simulink model "b_r309c_med"  (Simulink 6.2)
settings: Solver=ode45  StartTime=0.0  StopTime=1030.0  RelTol=1e-3
undefined symbols (not defined in the file): ant_bits, BEE2_usr, blockCountBits, blockRowBits, cmult_4bit_em
libraries: xbsIndex_r3 x2808, xps_library x97, casper_library x84
(part 7 of 20)

== system b_r309c_med/fmt_for_dram0/mk_4x32bit ==
  din : Inport  Port=1  LatchInput=off
  Concat3 : xbsIndex_r3/Concat  num_inputs=4  explicit_period=off  period=1  dbl_ovrd=off
  Convert{1..4} (4 alike) : xbsIndex_r3/Convert  arith_type="Signed  (2's comp)"  n_bits=32  bin_pt=0  quantization=Truncate  overflow=Wrap  latency=0  explicit_period=off  period=1  dbl_ovrd=off  show_param=off  inserted_by_tool=off  pipeline=off
      settings: xl_area=[0, 0, 0, 0, 0, 0, 0]
  Gateway Out{1..4,13..16} (8 alike) : xbsIndex_r3/Gateway Out  output_type=Double  nbits=8  bin_pt=6  arith_type=Boolean  quantization=Truncate  overflow=Wrap  hdl_port=off  timing_constraint=None  locs_specified=off  LOCs={}  needs_fixed_name=off  show_param=off
      settings: xl_area=[0, 0, 0, 0, 0, 0, 0]
  Reinterpret{,2,4,6} (4 alike) : xbsIndex_r3/Reinterpret  force_arith_type=on  arith_type=Unsigned  force_bin_pt=on  bin_pt=0  force_valid=on
  Reinterpret{1,3,5,7} (4 alike) : xbsIndex_r3/Reinterpret  force_arith_type=on  arith_type="Signed  (2's comp)"  force_bin_pt=on  bin_pt=0  force_valid=on
  Scope2 : Scope  NumInputPorts=8
      settings: YMin=0~0~0~0~0~0~0~0  YMax=20~20~20~20~20~20~20~20  SaveName=ScopeData3
  Slice10 : xbsIndex_r3/Slice  mode=Lower Bit Location + Width  nbits=(2*x_n_bits+1+x_int_bits)  bit1=0  base1=MSB of Input  bit0=2*(2*x_n_bits+1+x_int_bits)  base0=LSB of Input  boolean_output=off  explicit_period=off  period=1  dbl_ovrd=off
  Slice11 : xbsIndex_r3/Slice  mode=Lower Bit Location + Width  nbits=(2*x_n_bits+1+x_int_bits)  bit1=0  base1=MSB of Input  bit0=0  base0=LSB of Input  boolean_output=off  explicit_period=off  period=1  dbl_ovrd=off
  Slice12 : xbsIndex_r3/Slice  mode=Lower Bit Location + Width  nbits=(2*x_n_bits+1+x_int_bits)  bit1=0  base1=MSB of Input  bit0=(2*x_n_bits+1+x_int_bits)  base0=LSB of Input  boolean_output=off  explicit_period=off  period=1  dbl_ovrd=off
  Slice7 : xbsIndex_r3/Slice  mode=Lower Bit Location + Width  nbits=(2*x_n_bits+1+x_int_bits)  bit1=0  base1=MSB of Input  bit0=3*(2*x_n_bits+1+x_int_bits)  base0=LSB of Input  boolean_output=off  explicit_period=off  period=1  dbl_ovrd=off
  dout : Outport
  wires:
  Concat3/1 -> dout/1
  din/1 -> Slice12/1, Slice11/1, Slice10/1, Slice7/1
  Reinterpret6/1 -> Concat3/4
  Reinterpret4/1 -> Concat3/3
  Reinterpret2/1 -> Concat3/2
  Convert4/1 -> Reinterpret6/1, Gateway Out1/1
  Reinterpret7/1 -> Convert4/1, Gateway Out4/1
  Slice11/1 -> Reinterpret7/1
  Convert3/1 -> Reinterpret4/1, Gateway Out3/1
  Reinterpret5/1 -> Convert3/1, Gateway Out2/1
  Slice12/1 -> Reinterpret5/1
  Convert2/1 -> Reinterpret2/1, Gateway Out13/1
  Reinterpret3/1 -> Convert2/1, Gateway Out16/1
  Slice10/1 -> Reinterpret3/1
  Reinterpret/1 -> Concat3/1
  Convert1/1 -> Reinterpret/1, Gateway Out15/1
  Reinterpret1/1 -> Convert1/1, Gateway Out14/1
  Slice7/1 -> Reinterpret1/1
  Gateway Out14/1 -> Scope2/1
  Gateway Out15/1 -> Scope2/2
  Gateway Out16/1 -> Scope2/3
  Gateway Out13/1 -> Scope2/4
  Gateway Out2/1 -> Scope2/5
  Gateway Out3/1 -> Scope2/6
  Gateway Out4/1 -> Scope2/7
  Gateway Out1/1 -> Scope2/8

== system b_r309c_med/loopback0/fwft_fifo ==
  din : Inport  Port=1  LatchInput=off
  we : Inport  Port=2  LatchInput=off
  ack : Inport  Port=3  LatchInput=off
  Convert : xbsIndex_r3/Convert  Orientation=left  arith_type=Boolean  n_bits=1  bin_pt=0  quantization=Truncate  overflow=Wrap  latency=0  explicit_period=off  period=1  dbl_ovrd=off  show_param=off  inserted_by_tool=off  pipeline=off
      settings: xl_area=[0, 0, 0, 0, 0, 0, 0]
  FIFO : xbsIndex_r3/FIFO  depth=256  percent_nbits=1  store_only_valid=on  init_zero=on  explicit_period=off  period=1  rst=off  en=off  use_almost_empty=off  almost_empty_offset=6  use_almost_full=off  almost_full_offset=6  dbl_ovrd=off  show_param=off  mem_type=Block RAM  gen_core=off
      settings: xl_area=[0, 0, 0, 0, 0, 0, 0]
  Inverter1 : xbsIndex_r3/Inverter  latency=0  explicit_period=off  period=1  en=off  dbl_ovrd=off  show_param=off
      settings: xl_area=[0, 0, 0, 0, 0, 0, 0]
  Logical1 : xbsIndex_r3/Logical  logical_function=OR  inputs=2  precision=Full  arith_type=Unsigned  n_bits=8  bin_pt=2  align_bp=on  latency=0  explicit_period=off  period=1  en=off  dbl_ovrd=off  show_param=off
      settings: xl_area=[0, 0, 0, 0, 0, 0, 0]
  Register2 : xbsIndex_r3/Register  init=0  reg_only_valid=off  explicit_period=on  period=1  rst=off  en=on  out_en=off  dbl_ovrd=off  show_param=off
      settings: xl_area=[0, 0, 0, 0, 0, 0, 0]
  dout : Outport
  valid : Outport  Port=2
  wires:
  din/1 -> FIFO/1
  we/1 -> FIFO/2
  FIFO/1 -> dout/1
  FIFO/2 -> Register2/1
  Logical1/1 -> FIFO/3, Register2/2
  ack/1 -> Logical1/1
  Register2/1 -> Convert/1, Inverter1/1
  Convert/1 -> Logical1/2
  Inverter1/1 -> valid/1

== system b_r309c_med/loopback0/rollback_fifo ==
  din : Inport  Port=1  LatchInput=off
  we : Inport  Orientation=left  Port=2  LatchInput=off
  commit : Inport  Port=3  LatchInput=off
  discard : Inport  Port=4  LatchInput=off
  re : Inport  Port=5  LatchInput=off
  Constant5 : xbsIndex_r3/Constant  const=0  equ=P=C  arith_type=Boolean  n_bits=1  bin_pt=0  opselect=C  inp2=PCIN>>17  opr=+  inp1=P  carry=CIN  iostate=0  explicit_period=on  period=1  dbl_ovrd=off
  Delay1 : xbsIndex_r3/Delay  latency=1  reg_retiming=off  explicit_period=off  period=1  en=off  accept_only_valid=off  init_zero=on  dbl_ovrd=off  show_param=off
      settings: xl_area=[0, 0, 0, 0, 0, 0, 0]
  Dual Port RAM : xbsIndex_r3/Dual Port RAM  depth=2^depth_bits  initVector=0  write_mode_A=Read Before Write  write_mode_B=Read Before Write  latency=1  mem_collision=off  init_zero=on  explicit_period=off  period=1  dbl_ovrd=off  rst_a=off  init_a=0  rst_b=off  init_b=0  show_param=off  distributed_mem=off  use_rpm=off  gen_core=off
      settings: xl_area=[0, 0, 0, 0, 0, 0, 0]
  Inverter1 : xbsIndex_r3/Inverter  latency=0  explicit_period=off  period=1  en=off  dbl_ovrd=off  show_param=off
      settings: xl_area=[0, 0, 0, 0, 0, 0, 0]
  Inverter2 : xbsIndex_r3/Inverter  Orientation=up  latency=0  explicit_period=off  period=1  en=off  dbl_ovrd=off  show_param=off
      settings: xl_area=[0, 0, 0, 0, 0, 0, 0]
  Logical1 : xbsIndex_r3/Logical  logical_function=AND  inputs=2  precision=Full  arith_type=Unsigned  n_bits=8  bin_pt=2  align_bp=on  latency=0  explicit_period=off  period=1  en=off  dbl_ovrd=off  show_param=off
      settings: xl_area=[0, 0, 0, 0, 0, 0, 0]
  Logical3 : xbsIndex_r3/Logical  Orientation=left  logical_function=AND  inputs=2  precision=Full  arith_type=Unsigned  n_bits=8  bin_pt=2  align_bp=on  latency=0  explicit_period=off  period=1  en=off  dbl_ovrd=off  show_param=off
      settings: xl_area=[0, 0, 0, 0, 0, 0, 0]
  Logical4 : xbsIndex_r3/Logical  logical_function=AND  inputs=2  precision=Full  arith_type=Unsigned  n_bits=8  bin_pt=2  align_bp=on  latency=0  explicit_period=off  period=1  en=off  dbl_ovrd=off  show_param=off
      settings: xl_area=[0, 0, 0, 0, 0, 0, 0]
  Logical5 : xbsIndex_r3/Logical  logical_function=XOR  inputs=2  precision=Full  arith_type=Unsigned  n_bits=8  bin_pt=2  align_bp=on  latency=0  explicit_period=off  period=1  en=off  dbl_ovrd=off  show_param=off
      settings: xl_area=[0, 0, 0, 0, 0, 0, 0]
  Logical6 : xbsIndex_r3/Logical  logical_function=AND  inputs=2  precision=Full  arith_type=Unsigned  n_bits=8  bin_pt=2  align_bp=on  latency=0  explicit_period=off  period=1  en=off  dbl_ovrd=off  show_param=off
      settings: xl_area=[0, 0, 0, 0, 0, 0, 0]
  Relational1 : xbsIndex_r3/Relational  mode=a=b  latency=0  explicit_period=on  period=1  en=off  dbl_ovrd=off  show_param=off
      settings: xl_area=[0, 0, 0, 0, 0, 0, 0]
  Relational2 : xbsIndex_r3/Relational  mode=a=b  latency=0  explicit_period=on  period=1  en=off  dbl_ovrd=off  show_param=off
      settings: xl_area=[0, 0, 0, 0, 0, 0, 0]
  Slice : xbsIndex_r3/Slice  mode=Two Bit Locations  nbits=1  bit1=-1  base1=MSB of Input  bit0=0  base0=LSB of Input  boolean_output=off  explicit_period=off  period=1  dbl_ovrd=off
  Slice1 : xbsIndex_r3/Slice  mode=Upper Bit Location + Width  nbits=1  bit1=0  base1=MSB of Input  bit0=0  base0=LSB of Input  boolean_output=on  explicit_period=off  period=1  dbl_ovrd=off
  Slice2 : xbsIndex_r3/Slice  mode=Two Bit Locations  nbits=1  bit1=-1  base1=MSB of Input  bit0=0  base0=LSB of Input  boolean_output=off  explicit_period=off  period=1  dbl_ovrd=off
  Slice3 : xbsIndex_r3/Slice  mode=Upper Bit Location + Width  nbits=1  bit1=0  base1=MSB of Input  bit0=0  base0=LSB of Input  boolean_output=on  explicit_period=off  period=1  dbl_ovrd=off
  rd_cnt : xbsIndex_r3/Counter  cnt_type=Free Running  n_bits=depth_bits + 1  bin_pt=0  arith_type=Unsigned  start_count=0  cnt_to=Inf  cnt_by_val=1  operation=Up  explicit_period=on  period=1  load_pin=off  rst=off  en=on  dbl_ovrd=off  show_param=off  use_rpm=on  gen_core=off
      settings: xl_area=[0, 0, 0, 0, 0, 0, 0]
  set_cnt : Subsystem
  dout : Outport
  valid : Outport  Port=2
  wr_ack : Outport  Orientation=left  Port=3
  full : Outport  Port=4
  empty : Outport  Port=5
  wires:
  Relational2/1 -> Logical1/1
  Logical6/1 -> Inverter2/1, full/1
  Logical5/1 -> Logical6/1
  Relational1/1 -> Logical6/2
  Slice1/1 -> Logical5/2
  Slice3/1 -> Logical5/1
  Slice2/1 -> Relational1/1, Dual Port RAM/1
  din/1 -> Dual Port RAM/2, Dual Port RAM/5
  Slice/1 -> Relational1/2, Dual Port RAM/4
  set_cnt/2(cnt) -> Slice2/1, Slice3/1
  set_cnt/1(set_cnt) -> Relational2/1
  rd_cnt/1 -> Relational2/2, Slice1/1, Slice/1
  commit/1 -> set_cnt/1(set)
  Inverter2/1 -> Logical1/2, Logical3/1
  we/1 -> Logical3/2
  Logical3/1 -> wr_ack/1, Dual Port RAM/3, set_cnt/3(en)
  discard/1 -> set_cnt/2(undo)
  Constant5/1 -> Dual Port RAM/6
  Dual Port RAM/2 -> dout/1
  Logical1/1 -> Inverter1/1, empty/1
  Inverter1/1 -> Logical4/2
  re/1 -> Logical4/1
  Logical4/1 -> rd_cnt/1, Delay1/1
  Delay1/1 -> valid/1

== system b_r309c_med/mux_pkts0/state_mach ==
  note: state
  note: output
  gbe_valid : Inport  Port=1  LatchInput=off
  pkt_rdy : Inport  Port=2  LatchInput=off
  eof : Inport  Port=3  LatchInput=off
  Constant4 : xbsIndex_r3/Constant  const=1  equ=P=C  arith_type=Boolean  n_bits=1  bin_pt=0  opselect=C  inp2=PCIN>>17  opr=+  inp1=P  carry=CIN  iostate=0  explicit_period=on  period=1  dbl_ovrd=off
  Convert : xbsIndex_r3/Convert  arith_type=Boolean  n_bits=8  bin_pt=6  quantization=Truncate  overflow=Wrap  latency=0  explicit_period=off  period=1  dbl_ovrd=off  show_param=off  inserted_by_tool=off  pipeline=off
      settings: xl_area=[0, 0, 0, 0, 0, 0, 0]
  Inverter : xbsIndex_r3/Inverter  latency=0  explicit_period=off  period=1  en=off  dbl_ovrd=off  show_param=off
      settings: xl_area=[0, 0, 0, 0, 0, 0, 0]
  Inverter1 : xbsIndex_r3/Inverter  Orientation=left  latency=0  explicit_period=off  period=1  en=off  dbl_ovrd=off  show_param=off
      settings: xl_area=[0, 0, 0, 0, 0, 0, 0]
  Inverter2 : xbsIndex_r3/Inverter  latency=0  explicit_period=off  period=1  en=off  dbl_ovrd=off  show_param=off
      settings: xl_area=[0, 0, 0, 0, 0, 0, 0]
  Logical1 : xbsIndex_r3/Logical  logical_function=AND  inputs=2  precision=Full  arith_type=Unsigned  n_bits=8  bin_pt=2  align_bp=on  latency=0  explicit_period=off  period=1  en=off  dbl_ovrd=off  show_param=off
      settings: xl_area=[0, 0, 0, 0, 0, 0, 0]
  Logical2 : xbsIndex_r3/Logical  logical_function=OR  inputs=2  precision=Full  arith_type=Unsigned  n_bits=8  bin_pt=2  align_bp=on  latency=0  explicit_period=off  period=1  en=off  dbl_ovrd=off  show_param=off
      settings: xl_area=[0, 0, 0, 0, 0, 0, 0]
  Logical3 : xbsIndex_r3/Logical  logical_function=AND  inputs=2  precision=Full  arith_type=Unsigned  n_bits=8  bin_pt=2  align_bp=on  latency=0  explicit_period=off  period=1  en=off  dbl_ovrd=off  show_param=off
      settings: xl_area=[0, 0, 0, 0, 0, 0, 0]
  Logical4 : xbsIndex_r3/Logical  logical_function=AND  inputs=2  precision=Full  arith_type=Unsigned  n_bits=8  bin_pt=2  align_bp=on  latency=0  explicit_period=off  period=1  en=off  dbl_ovrd=off  show_param=off
      settings: xl_area=[0, 0, 0, 0, 0, 0, 0]
  Register1 : xbsIndex_r3/Register  init=0  reg_only_valid=off  explicit_period=on  period=1  rst=on  en=on  out_en=off  dbl_ovrd=off  show_param=off
      settings: xl_area=[0, 0, 0, 0, 0, 0, 0]
  Register2 : xbsIndex_r3/Register  init=0  reg_only_valid=off  explicit_period=on  period=1  rst=off  en=on  out_en=off  dbl_ovrd=off  show_param=off
      settings: xl_area=[0, 0, 0, 0, 0, 0, 0]
  gbe_ack : Outport
  loop_ack : Outport  Port=2
  state : Outport  Port=3
  wires:
  Register1/1 -> Convert/1
  Constant4/1 -> Register1/1
  Logical2/1 -> Logical3/2, Register1/3
  Logical3/1 -> Register2/2
  Inverter2/1 -> Register2/1
  gbe_valid/1 -> Logical2/1
  Register2/1 -> Inverter/1, Logical4/2
  Inverter1/1 -> Logical3/1
  eof/1 -> Register1/2
  Inverter/1 -> Logical1/2
  Logical1/1 -> loop_ack/1
  Logical4/1 -> gbe_ack/1
  pkt_rdy/1 -> Logical2/2, Inverter2/1
  Convert/1 -> state/1, Logical1/1, Logical4/1, Inverter1/1

== system b_r309c_med/out_mon0/stopwatch ==
  stop : Inport  Port=1  LatchInput=off
  start : Inport  Port=2  LatchInput=off
  reset : Inport  Port=3  LatchInput=off
  count : Inport  Port=4  LatchInput=off
  Constant1 : xbsIndex_r3/Constant  const=1  equ=P=C  arith_type=Boolean  n_bits=1  bin_pt=0  opselect=C  inp2=PCIN>>17  opr=+  inp1=P  carry=CIN  iostate=0  explicit_period=on  period=1  dbl_ovrd=off
  Constant8 : xbsIndex_r3/Constant  const=1  equ=P=C  arith_type=Boolean  n_bits=1  bin_pt=0  opselect=C  inp2=PCIN>>17  opr=+  inp1=P  carry=CIN  iostate=0  explicit_period=on  period=1  dbl_ovrd=off
  Counter1 : xbsIndex_r3/Counter  cnt_type=Free Running  n_bits=32  bin_pt=0  arith_type=Unsigned  start_count=0  cnt_to=Inf  cnt_by_val=1  operation=Up  explicit_period=off  period=1  load_pin=off  rst=on  en=on  dbl_ovrd=off  show_param=off  use_rpm=on  gen_core=off
      settings: xl_area=[0, 0, 0, 0, 0, 0, 0]
  Logical : xbsIndex_r3/Logical  logical_function=AND  inputs=3  precision=Full  arith_type=Unsigned  n_bits=8  bin_pt=2  align_bp=on  latency=0  explicit_period=off  period=1  en=off  dbl_ovrd=off  show_param=off
      settings: xl_area=[0, 0, 0, 0, 0, 0, 0]
  Register1 : xbsIndex_r3/Register  init=0  reg_only_valid=off  explicit_period=off  period=1  rst=on  en=on  out_en=off  dbl_ovrd=off  show_param=off
      settings: xl_area=[0, 0, 0, 0, 0, 0, 0]
  Register3 : xbsIndex_r3/Register  init=0  reg_only_valid=off  explicit_period=off  period=1  rst=on  en=on  out_en=off  dbl_ovrd=off  show_param=off
      settings: xl_area=[0, 0, 0, 0, 0, 0, 0]
  count_out : Outport
  wires:
  Constant8/1 -> Register3/1
  Counter1/1 -> count_out/1
  Constant1/1 -> Register1/1
  start/1 -> Register1/3
  reset/1 -> Counter1/1, Register1/2, Register3/3
  Logical/1 -> Counter1/2
  Register3/1 -> Logical/1
  Register1/1 -> Logical/2
  stop/1 -> Register3/2
  count/1 -> Logical/3

== system b_r309c_med/out_mon0/x_eng_cntr ==
  note: n_ants*(n_ants+1)/2 * n_chans/n_xeng-1
  acc_in : Inport  Port=1  LatchInput=off
  valid_in : Inport  Port=2  LatchInput=off
  sync_in : Inport  Port=3  LatchInput=off
  Constant9 : xbsIndex_r3/Constant  Orientation=left  const=n_ants*(n_ants+1)/2 * n_chans/n_xeng-1  equ=P=C  arith_type=Unsigned  n_bits=32  bin_pt=0  opselect=C  inp2=PCIN>>17  opr=+  inp1=P  carry=CIN  iostate=0  explicit_period=on  period=1  dbl_ovrd=off
  Logical6 : xbsIndex_r3/Logical  logical_function=OR  inputs=2  precision=Full  arith_type=Unsigned  n_bits=8  bin_pt=2  align_bp=on  latency=0  explicit_period=on  period=1  en=off  dbl_ovrd=off  show_param=off
      settings: xl_area=[0, 0, 0, 0, 0, 0, 0]
  Relational : xbsIndex_r3/Relational  Orientation=left  mode=a=b  latency=1  explicit_period=on  period=1  en=off  dbl_ovrd=off  show_param=off
      settings: xl_area=[0, 0, 0, 0, 0, 0, 0]
  window_cntr : xbsIndex_r3/Counter  cnt_type=Free Running  n_bits=32  bin_pt=0  arith_type=Unsigned  start_count=0  cnt_to=Inf  cnt_by_val=1  operation=Up  explicit_period=on  period=1  load_pin=off  rst=on  en=on  dbl_ovrd=off  show_param=off  use_rpm=on  gen_core=off
      settings: xl_area=[0, 0, 0, 0, 0, 0, 0]
  acc_out : Outport
  valid_out : Outport  Port=2
  sync_out : Outport  Port=3
  window_position : Outport  Port=4
  wires:
  Logical6/1 -> window_cntr/1
  Constant9/1 -> Relational/2
  window_cntr/1 -> Relational/1, window_position/1
  sync_in/1 -> Logical6/2, sync_out/1
  valid_in/1 -> window_cntr/2, valid_out/1
  Relational/1 -> Logical6/1
  acc_in/1 -> acc_out/1

== system b_r309c_med/pack_it0/neg_edge_delay ==
  in : Inport  Port=1  LatchInput=off
  Constant5 : xbsIndex_r3/Constant  const=pulse_len  equ=P=C  arith_type=Unsigned  n_bits=bits  bin_pt=0  opselect=C  inp2=PCIN>>17  opr=+  inp1=P  carry=CIN  iostate=0  explicit_period=off  period=1  dbl_ovrd=off
  Counter3 : xbsIndex_r3/Counter  cnt_type=Free Running  n_bits=bits  bin_pt=0  arith_type=Unsigned  start_count=0  cnt_to=1023  cnt_by_val=1  operation=Up  explicit_period=on  period=1  load_pin=off  rst=on  en=on  dbl_ovrd=off  show_param=off  use_rpm=on  gen_core=off
      settings: xl_area=[0, 0, 0, 0, 0, 0, 0]
  Relational5 : xbsIndex_r3/Relational  mode=a!=b  latency=0  explicit_period=off  period=1  en=off  dbl_ovrd=off  show_param=off
      settings: xl_area=[0, 0, 0, 0, 0, 0, 0]
  out : Outport
  wires:
  Relational5/1 -> out/1, Counter3/2
  Constant5/1 -> Relational5/2
  Counter3/1 -> Relational5/1
  in/1 -> Counter3/1

== system b_r309c_med/pack_it0/oob_decode ==
  note: if we're not getting a header or ant_levels data,
      | then it must be ordinary data
  valid_in : Inport  Orientation=up  Port=1  LatchInput=off
  oob_in : Inport  Port=2  LatchInput=off
  Inverter1 : xbsIndex_r3/Inverter  latency=0  explicit_period=off  period=1  en=off  dbl_ovrd=off  show_param=off
      settings: xl_area=[0, 0, 0, 0, 0, 0, 0]
  Inverter5 : xbsIndex_r3/Inverter  latency=0  explicit_period=off  period=1  en=off  dbl_ovrd=off  show_param=off
      settings: xl_area=[0, 0, 0, 0, 0, 0, 0]
  Logical1 : xbsIndex_r3/Logical  logical_function=AND  inputs=3  precision=Full  arith_type=Unsigned  n_bits=8  bin_pt=2  align_bp=on  latency=0  explicit_period=off  period=1  en=off  dbl_ovrd=off  show_param=off
      settings: xl_area=[0, 0, 0, 0, 0, 0, 0]
  Logical{2..4,7} (4 alike) : xbsIndex_r3/Logical  logical_function=AND  inputs=2  precision=Full  arith_type=Unsigned  n_bits=8  bin_pt=2  align_bp=on  latency=0  explicit_period=off  period=1  en=off  dbl_ovrd=off  show_param=off
      settings: xl_area=[0, 0, 0, 0, 0, 0, 0]
  Slice1 : xbsIndex_r3/Slice  mode=Lower Bit Location + Width  nbits=1  bit1=0  base1=MSB of Input  bit0=2  base0=LSB of Input  boolean_output=on  explicit_period=off  period=1  dbl_ovrd=off
  Slice2 : xbsIndex_r3/Slice  mode=Lower Bit Location + Width  nbits=1  bit1=0  base1=MSB of Input  bit0=0  base0=LSB of Input  boolean_output=on  explicit_period=off  period=1  dbl_ovrd=off
  Slice3 : xbsIndex_r3/Slice  mode=Lower Bit Location + Width  nbits=1  bit1=0  base1=MSB of Input  bit0=1  base0=LSB of Input  boolean_output=on  explicit_period=off  period=1  dbl_ovrd=off
  Slice6 : xbsIndex_r3/Slice  mode=Lower Bit Location + Width  nbits=1  bit1=0  base1=MSB of Input  bit0=3  base0=LSB of Input  boolean_output=on  explicit_period=off  period=1  dbl_ovrd=off
  Slice8 : xbsIndex_r3/Slice  mode=Lower Bit Location + Width  nbits=1  bit1=0  base1=MSB of Input  bit0=4  base0=LSB of Input  boolean_output=on  explicit_period=off  period=1  dbl_ovrd=off
  packet_data : Outport
  mrst : Outport  Port=2
  sync : Outport  Port=3
  ant_levels : Outport  Port=4
  eof : Outport  Port=5
  header : Outport  Port=6
  wires:
  Slice8/1 -> mrst/1
  oob_in/1 -> Slice3/1, Slice1/1, Slice6/1, Slice8/1, Slice2/1
  valid_in/1 -> Logical3/2, Logical2/2, Logical7/2, Logical1/2, Logical4/2
  Logical1/1 -> packet_data/1
  Inverter5/1 -> Logical1/1
  Logical7/1 -> ant_levels/1
  Slice1/1 -> Logical2/1
  Logical2/1 -> eof/1
  Slice6/1 -> Logical7/1, Inverter5/1
  Slice2/1 -> Logical3/1, Inverter1/1
  Logical3/1 -> header/1
  Inverter1/1 -> Logical1/3
  Slice3/1 -> Logical4/1
  Logical4/1 -> sync/1

== system b_r309c_med/pack_it1/neg_edge_delay ==
  in : Inport  Port=1  LatchInput=off
  Constant5 : xbsIndex_r3/Constant  const=pulse_len  equ=P=C  arith_type=Unsigned  n_bits=bits  bin_pt=0  opselect=C  inp2=PCIN>>17  opr=+  inp1=P  carry=CIN  iostate=0  explicit_period=off  period=1  dbl_ovrd=off
  Counter3 : xbsIndex_r3/Counter  cnt_type=Free Running  n_bits=bits  bin_pt=0  arith_type=Unsigned  start_count=0  cnt_to=1023  cnt_by_val=1  operation=Up  explicit_period=on  period=1  load_pin=off  rst=on  en=on  dbl_ovrd=off  show_param=off  use_rpm=on  gen_core=off
      settings: xl_area=[0, 0, 0, 0, 0, 0, 0]
  Relational5 : xbsIndex_r3/Relational  mode=a!=b  latency=0  explicit_period=off  period=1  en=off  dbl_ovrd=off  show_param=off
      settings: xl_area=[0, 0, 0, 0, 0, 0, 0]
  out : Outport
  wires:
  Relational5/1 -> out/1, Counter3/2
  Constant5/1 -> Relational5/2
  Counter3/1 -> Relational5/1
  in/1 -> Counter3/1

== system b_r309c_med/pack_it1/oob_decode ==
  note: if we're not getting a header or ant_levels data,
      | then it must be ordinary data
  valid_in : Inport  Orientation=up  Port=1  LatchInput=off
  oob_in : Inport  Port=2  LatchInput=off
  Inverter1 : xbsIndex_r3/Inverter  latency=0  explicit_period=off  period=1  en=off  dbl_ovrd=off  show_param=off
      settings: xl_area=[0, 0, 0, 0, 0, 0, 0]
  Inverter5 : xbsIndex_r3/Inverter  latency=0  explicit_period=off  period=1  en=off  dbl_ovrd=off  show_param=off
      settings: xl_area=[0, 0, 0, 0, 0, 0, 0]
  Logical1 : xbsIndex_r3/Logical  logical_function=AND  inputs=3  precision=Full  arith_type=Unsigned  n_bits=8  bin_pt=2  align_bp=on  latency=0  explicit_period=off  period=1  en=off  dbl_ovrd=off  show_param=off
      settings: xl_area=[0, 0, 0, 0, 0, 0, 0]
  Logical{2..4,7} (4 alike) : xbsIndex_r3/Logical  logical_function=AND  inputs=2  precision=Full  arith_type=Unsigned  n_bits=8  bin_pt=2  align_bp=on  latency=0  explicit_period=off  period=1  en=off  dbl_ovrd=off  show_param=off
      settings: xl_area=[0, 0, 0, 0, 0, 0, 0]
  Slice1 : xbsIndex_r3/Slice  mode=Lower Bit Location + Width  nbits=1  bit1=0  base1=MSB of Input  bit0=2  base0=LSB of Input  boolean_output=on  explicit_period=off  period=1  dbl_ovrd=off
  Slice2 : xbsIndex_r3/Slice  mode=Lower Bit Location + Width  nbits=1  bit1=0  base1=MSB of Input  bit0=0  base0=LSB of Input  boolean_output=on  explicit_period=off  period=1  dbl_ovrd=off
  Slice3 : xbsIndex_r3/Slice  mode=Lower Bit Location + Width  nbits=1  bit1=0  base1=MSB of Input  bit0=1  base0=LSB of Input  boolean_output=on  explicit_period=off  period=1  dbl_ovrd=off
  Slice6 : xbsIndex_r3/Slice  mode=Lower Bit Location + Width  nbits=1  bit1=0  base1=MSB of Input  bit0=3  base0=LSB of Input  boolean_output=on  explicit_period=off  period=1  dbl_ovrd=off
  Slice8 : xbsIndex_r3/Slice  mode=Lower Bit Location + Width  nbits=1  bit1=0  base1=MSB of Input  bit0=4  base0=LSB of Input  boolean_output=on  explicit_period=off  period=1  dbl_ovrd=off
  packet_data : Outport
  mrst : Outport  Port=2
  sync : Outport  Port=3
  ant_levels : Outport  Port=4
  eof : Outport  Port=5
  header : Outport  Port=6
  wires:
  Slice8/1 -> mrst/1
  oob_in/1 -> Slice3/1, Slice1/1, Slice6/1, Slice8/1, Slice2/1
  valid_in/1 -> Logical3/2, Logical2/2, Logical7/2, Logical1/2, Logical4/2
  Logical1/1 -> packet_data/1
  Inverter5/1 -> Logical1/1
  Logical7/1 -> ant_levels/1
  Slice1/1 -> Logical2/1
  Logical2/1 -> eof/1
  Slice6/1 -> Logical7/1, Inverter5/1
  Slice2/1 -> Logical3/1, Inverter1/1
  Logical3/1 -> header/1
  Inverter1/1 -> Logical1/3
  Slice3/1 -> Logical4/1
  Logical4/1 -> sync/1

== system b_r309c_med/pulse_ext1/freeze_cntr ==
  en : Inport  Port=1  LatchInput=off
  rst : Inport  Port=2  LatchInput=off
  Constant5 : xbsIndex_r3/Constant  const=2^CounterBits - 1  equ=P=C  arith_type=Unsigned  n_bits=CounterBits  bin_pt=0  opselect=C  inp2=PCIN>>17  opr=+  inp1=P  carry=CIN  iostate=0  explicit_period=off  period=1  dbl_ovrd=off
  Counter3 : xbsIndex_r3/Counter  cnt_type=Free Running  n_bits=CounterBits  bin_pt=0  arith_type=Unsigned  start_count=0  cnt_to=1023  cnt_by_val=1  operation=Up  explicit_period=on  period=1  load_pin=off  rst=on  en=on  dbl_ovrd=off  show_param=off  use_rpm=on  gen_core=off
      settings: xl_area=[0, 0, 0, 0, 0, 0, 0]
  Inverter : xbsIndex_r3/Inverter  latency=0  explicit_period=off  period=1  en=off  dbl_ovrd=off  show_param=off
      settings: xl_area=[0, 0, 0, 0, 0, 0, 0]
  Logical1 : xbsIndex_r3/Logical  logical_function=AND  inputs=2  precision=Full  arith_type=Unsigned  n_bits=8  bin_pt=2  align_bp=on  latency=0  explicit_period=off  period=1  en=off  dbl_ovrd=off  show_param=off
      settings: xl_area=[0, 0, 0, 0, 0, 0, 0]
  Logical5 : xbsIndex_r3/Logical  logical_function=AND  inputs=2  precision=Full  arith_type=Unsigned  n_bits=8  bin_pt=2  align_bp=on  latency=0  explicit_period=off  period=1  en=off  dbl_ovrd=off  show_param=off
      settings: xl_area=[0, 0, 0, 0, 0, 0, 0]
  Relational5 : xbsIndex_r3/Relational  mode=a!=b  latency=0  explicit_period=off  period=1  en=off  dbl_ovrd=off  show_param=off
      settings: xl_area=[0, 0, 0, 0, 0, 0, 0]
  addr : Outport
  we : Outport  Port=2
  wires:
  rst/1 -> Counter3/1, Inverter/1
  Logical5/1 -> Counter3/2, Logical1/2
  en/1 -> Logical5/1
  Relational5/1 -> Logical5/2
  Constant5/1 -> Relational5/2
  Counter3/1 -> Relational5/1, addr/1
  Inverter/1 -> Logical1/1
  Logical1/1 -> we/1

== system b_r309c_med/pulse_ext1/posedge ==
  In : Inport  Port=1  LatchInput=off
  Delay : xbsIndex_r3/Delay  latency=1  reg_retiming=off  explicit_period=off  period=1  en=off  accept_only_valid=off  init_zero=on  dbl_ovrd=off  show_param=off
      settings: xl_area=[0, 0, 0, 0, 0, 0, 0]
  Inverter : xbsIndex_r3/Inverter  latency=0  explicit_period=off  period=1  en=off  dbl_ovrd=off  show_param=off
      settings: xl_area=[0, 0, 0, 0, 0, 0, 0]
  Logical : xbsIndex_r3/Logical  logical_function=AND  inputs=2  precision=Full  arith_type=Unsigned  n_bits=8  bin_pt=2  align_bp=on  latency=0  explicit_period=off  period=1  en=off  dbl_ovrd=off  show_param=off
      settings: xl_area=[0, 0, 0, 0, 0, 0, 0]
  Out : Outport
  wires:
  Delay/1 -> Inverter/1
  Inverter/1 -> Logical/1
  In/1 -> Delay/1, Logical/2
  Logical/1 -> Out/1

== system b_r309c_med/pulse_ext2/freeze_cntr ==
  en : Inport  Port=1  LatchInput=off
  rst : Inport  Port=2  LatchInput=off
  Constant5 : xbsIndex_r3/Constant  const=2^CounterBits - 1  equ=P=C  arith_type=Unsigned  n_bits=CounterBits  bin_pt=0  opselect=C  inp2=PCIN>>17  opr=+  inp1=P  carry=CIN  iostate=0  explicit_period=off  period=1  dbl_ovrd=off
  Counter3 : xbsIndex_r3/Counter  cnt_type=Free Running  n_bits=CounterBits  bin_pt=0  arith_type=Unsigned  start_count=0  cnt_to=1023  cnt_by_val=1  operation=Up  explicit_period=on  period=1  load_pin=off  rst=on  en=on  dbl_ovrd=off  show_param=off  use_rpm=on  gen_core=off
      settings: xl_area=[0, 0, 0, 0, 0, 0, 0]
  Inverter : xbsIndex_r3/Inverter  latency=0  explicit_period=off  period=1  en=off  dbl_ovrd=off  show_param=off
      settings: xl_area=[0, 0, 0, 0, 0, 0, 0]
  Logical1 : xbsIndex_r3/Logical  logical_function=AND  inputs=2  precision=Full  arith_type=Unsigned  n_bits=8  bin_pt=2  align_bp=on  latency=0  explicit_period=off  period=1  en=off  dbl_ovrd=off  show_param=off
      settings: xl_area=[0, 0, 0, 0, 0, 0, 0]
  Logical5 : xbsIndex_r3/Logical  logical_function=AND  inputs=2  precision=Full  arith_type=Unsigned  n_bits=8  bin_pt=2  align_bp=on  latency=0  explicit_period=off  period=1  en=off  dbl_ovrd=off  show_param=off
      settings: xl_area=[0, 0, 0, 0, 0, 0, 0]
  Relational5 : xbsIndex_r3/Relational  mode=a!=b  latency=0  explicit_period=off  period=1  en=off  dbl_ovrd=off  show_param=off
      settings: xl_area=[0, 0, 0, 0, 0, 0, 0]
  addr : Outport
  we : Outport  Port=2
  wires:
  rst/1 -> Counter3/1, Inverter/1
  Logical5/1 -> Counter3/2, Logical1/2
  en/1 -> Logical5/1
  Relational5/1 -> Logical5/2
  Constant5/1 -> Relational5/2
  Counter3/1 -> Relational5/1, addr/1
  Inverter/1 -> Logical1/1
  Logical1/1 -> we/1

== system b_r309c_med/pulse_ext2/posedge ==
  In : Inport  Port=1  LatchInput=off
  Delay : xbsIndex_r3/Delay  latency=1  reg_retiming=off  explicit_period=off  period=1  en=off  accept_only_valid=off  init_zero=on  dbl_ovrd=off  show_param=off
      settings: xl_area=[0, 0, 0, 0, 0, 0, 0]
  Inverter : xbsIndex_r3/Inverter  latency=0  explicit_period=off  period=1  en=off  dbl_ovrd=off  show_param=off
      settings: xl_area=[0, 0, 0, 0, 0, 0, 0]
  Logical : xbsIndex_r3/Logical  logical_function=AND  inputs=2  precision=Full  arith_type=Unsigned  n_bits=8  bin_pt=2  align_bp=on  latency=0  explicit_period=off  period=1  en=off  dbl_ovrd=off  show_param=off
      settings: xl_area=[0, 0, 0, 0, 0, 0, 0]
  Out : Outport
  wires:
  Delay/1 -> Inverter/1
  Inverter/1 -> Logical/1
  In/1 -> Delay/1, Logical/2
  Logical/1 -> Out/1

== system b_r309c_med/snap_acc0/posedge ==
  In : Inport  Port=1  LatchInput=off
  Delay : xbsIndex_r3/Delay  latency=1  reg_retiming=off  explicit_period=off  period=1  en=off  accept_only_valid=off  init_zero=on  dbl_ovrd=off  show_param=off
      settings: xl_area=[0, 0, 0, 0, 0, 0, 0]
  Inverter : xbsIndex_r3/Inverter  latency=0  explicit_period=off  period=1  en=off  dbl_ovrd=off  show_param=off
      settings: xl_area=[0, 0, 0, 0, 0, 0, 0]
  Logical : xbsIndex_r3/Logical  logical_function=AND  inputs=2  precision=Full  arith_type=Unsigned  n_bits=8  bin_pt=2  align_bp=on  latency=0  explicit_period=off  period=1  en=off  dbl_ovrd=off  show_param=off
      settings: xl_area=[0, 0, 0, 0, 0, 0, 0]
  Out : Outport
  wires:
  Logical/1 -> Out/1
  In/1 -> Logical/2, Delay/1
  Inverter/1 -> Logical/1
  Delay/1 -> Inverter/1

== system b_r309c_med/win_x_engine0/auto_tap ==
  a_del : Inport  Port=1  LatchInput=off
  a_ndel : Inport  Port=2  LatchInput=off
  a_loop : Inport  Port=3  LatchInput=off
  acc_in : Inport  Port=4  LatchInput=off
  valid_in : Inport  Port=5  LatchInput=off
  sync_in : Inport  Port=6  LatchInput=off
  a_loop_delay : Subsystem  BlockChoice=delay_bram
      link override delay_bram: DelayLen=(acc_len - 1)*ceil(n_ants/2) + ceil(n_ants/2)-floor(n_ants/2)  bram_latency=bram_latency
      link override delay_bram/Constant2: equ=P=C
      settings: AttributesFormatString=%<BlockChoice>  TemplateBlock=casper_library/Delays/delay  MemberBlocks=delay_bram,delay_slr
  dual_pol_cmac : Subsystem
  sync_delay : casper_library/Delays/sync_delay  DelayLen=add_latency + mult_latency + acc_len + floor(n_ants/2 + 1) + 1
      link override Constant: equ=P=C
      link override Constant1: equ=P=C
      link override Constant2: equ=P=C
      link override Constant3: equ=P=C
  a_del_out : Outport
  a_ndel_out : Outport  Port=2
  a_end_out : Outport  Port=3
  acc_out : Outport  Port=4
  valid_out : Outport  Port=5
  rst_out : Outport  Port=6
  sync_out : Outport  Port=7
  wires:
  sync_in/1 -> sync_delay/1, dual_pol_cmac/4(sync), rst_out/1
  a_del/1 -> dual_pol_cmac/1(a1), a_del_out/1
  dual_pol_cmac/1(acc_out) -> acc_out/1
  acc_in/1 -> dual_pol_cmac/3(acc_in)
  dual_pol_cmac/2(valid_out) -> valid_out/1
  valid_in/1 -> dual_pol_cmac/5(valid_in)
  a_ndel/1 -> dual_pol_cmac/2(a2), a_ndel_out/1
  a_loop/1 -> a_loop_delay/1(In1)
  a_loop_delay/1(Out1) -> a_end_out/1
  sync_delay/1 -> sync_out/1

== system b_r309c_med/win_x_engine0/baseline_tap1 ==
  a_del : Inport  Port=1  LatchInput=off
  a_ndel : Inport  Port=2  LatchInput=off
  a_end : Inport  Port=3  LatchInput=off
  acc_in : Inport  Port=4  LatchInput=off
  valid_in : Inport  Port=5  LatchInput=off
  rst : Inport  Port=6  LatchInput=off
  sync1 : Inport  Port=7  LatchInput=off
  Constant : xbsIndex_r3/Constant  const=ant_sep * acc_len  equ=P=C  arith_type=Unsigned  n_bits=ant_bits + bit_growth  bin_pt=0  opselect=C  inp2=PCIN>>17  opr=+  inp1=P  carry=CIN  iostate=0  explicit_period=off  period=1  dbl_ovrd=off
  Convert : xbsIndex_r3/Convert  arith_type=Unsigned  n_bits=1  bin_pt=0  quantization=Truncate  overflow=Wrap  latency=0  explicit_period=off  period=1  dbl_ovrd=off  show_param=off  inserted_by_tool=off  pipeline=off
      settings: xl_area=[0, 0, 0, 0, 0, 0, 0]
  Counter : xbsIndex_r3/Counter  cnt_type=Count Limited  n_bits=ant_bits + bit_growth  bin_pt=0  arith_type=Unsigned  start_count=0  cnt_to=n_ants * acc_len - 1  cnt_by_val=1  operation=Up  explicit_period=off  period=1  load_pin=off  rst=on  en=off  dbl_ovrd=off  show_param=off  use_rpm=on  gen_core=off
      settings: xl_area=[0, 0, 0, 0, 0, 0, 0]
  Delay1 : xbsIndex_r3/Delay  latency=1  reg_retiming=off  explicit_period=off  period=1  en=off  accept_only_valid=off  init_zero=on  dbl_ovrd=off  show_param=off
      settings: xl_area=[0, 0, 0, 0, 0, 0, 0]
  Delay3 : xbsIndex_r3/Delay  latency=1  reg_retiming=off  explicit_period=off  period=1  en=off  accept_only_valid=off  init_zero=on  dbl_ovrd=off  show_param=off
      settings: xl_area=[0, 0, 0, 0, 0, 0, 0]
  Delay7 : xbsIndex_r3/Delay  latency=1  reg_retiming=off  explicit_period=on  period=1  en=off  accept_only_valid=off  init_zero=on  dbl_ovrd=off  show_param=off
      settings: xl_area=[0, 0, 0, 0, 0, 0, 0]
  Delay8 : xbsIndex_r3/Delay  latency=1  reg_retiming=off  explicit_period=on  period=1  en=off  accept_only_valid=off  init_zero=on  dbl_ovrd=off  show_param=off
      settings: xl_area=[0, 0, 0, 0, 0, 0, 0]
  Mux : xbsIndex_r3/Mux  inputs=2  precision=Full  arith_type="Signed  (2's comp)"  n_bits=8  bin_pt=2  quantization=Truncate  overflow=Wrap  latency=1  explicit_period=off  period=1  en=off  dbl_ovrd=off  show_param=off  mux_type=off  use_rpm=off  gen_core=off
      settings: xl_area=[0, 0, 0, 0, 0, 0, 0]
  Relational : xbsIndex_r3/Relational  mode=a<b  latency=0  explicit_period=off  period=1  en=off  dbl_ovrd=off  show_param=off
      settings: xl_area=[0, 0, 0, 0, 0, 0, 0]
  delay : Subsystem  BlockChoice=delay_bram
      link override delay_bram: DelayLen=acc_len  bram_latency=bram_latency
      link override delay_bram/Constant2: equ=P=C
      link override delay_slr: DelayLen=acc_len
      settings: AttributesFormatString=%<BlockChoice>  TemplateBlock=casper_library/Delays/delay  MemberBlocks=delay_bram,delay_slr
  dual_pol_cmac : Subsystem
  a_del_out : Outport
  a_ndel_out : Outport  Port=2
  a_end_out : Outport  Port=3
  acc_out : Outport  Port=4
  valid_out : Outport  Port=5
  rst_out : Outport  Port=6
  sync_out : Outport  Port=7
  wires:
  delay/1(Out1) -> Delay3/1
  Mux/1 -> dual_pol_cmac/2(a2)
  Counter/1 -> Relational/1
  Constant/1 -> Relational/2
  Relational/1 -> Convert/1
  Convert/1 -> Mux/1
  rst/1 -> Delay1/1, Counter/1
  a_del/1 -> delay/1(In1)
  dual_pol_cmac/1(acc_out) -> acc_out/1
  acc_in/1 -> dual_pol_cmac/3(acc_in)
  dual_pol_cmac/2(valid_out) -> valid_out/1
  valid_in/1 -> dual_pol_cmac/5(valid_in)
  a_ndel/1 -> Mux/2, Delay7/1
  a_end/1 -> Mux/3, Delay8/1
  Delay3/1 -> dual_pol_cmac/1(a1), a_del_out/1
  Delay7/1 -> a_ndel_out/1
  Delay8/1 -> a_end_out/1
  Delay1/1 -> dual_pol_cmac/4(sync), rst_out/1
  sync1/1 -> sync_out/1

== system b_r309c_med/win_x_engine0/baseline_tap2 ==
  a_del : Inport  Port=1  LatchInput=off
  a_ndel : Inport  Port=2  LatchInput=off
  a_end : Inport  Port=3  LatchInput=off
  acc_in : Inport  Port=4  LatchInput=off
  valid_in : Inport  Port=5  LatchInput=off
  rst : Inport  Port=6  LatchInput=off
  sync1 : Inport  Port=7  LatchInput=off
  Constant : xbsIndex_r3/Constant  const=ant_sep * acc_len  equ=P=C  arith_type=Unsigned  n_bits=ant_bits + bit_growth  bin_pt=0  opselect=C  inp2=PCIN>>17  opr=+  inp1=P  carry=CIN  iostate=0  explicit_period=off  period=1  dbl_ovrd=off
  Convert : xbsIndex_r3/Convert  arith_type=Unsigned  n_bits=1  bin_pt=0  quantization=Truncate  overflow=Wrap  latency=0  explicit_period=off  period=1  dbl_ovrd=off  show_param=off  inserted_by_tool=off  pipeline=off
      settings: xl_area=[0, 0, 0, 0, 0, 0, 0]
  Counter : xbsIndex_r3/Counter  cnt_type=Count Limited  n_bits=ant_bits + bit_growth  bin_pt=0  arith_type=Unsigned  start_count=0  cnt_to=n_ants * acc_len - 1  cnt_by_val=1  operation=Up  explicit_period=off  period=1  load_pin=off  rst=on  en=off  dbl_ovrd=off  show_param=off  use_rpm=on  gen_core=off
      settings: xl_area=[0, 0, 0, 0, 0, 0, 0]
  Delay1 : xbsIndex_r3/Delay  latency=1  reg_retiming=off  explicit_period=off  period=1  en=off  accept_only_valid=off  init_zero=on  dbl_ovrd=off  show_param=off
      settings: xl_area=[0, 0, 0, 0, 0, 0, 0]
  Delay3 : xbsIndex_r3/Delay  latency=1  reg_retiming=off  explicit_period=off  period=1  en=off  accept_only_valid=off  init_zero=on  dbl_ovrd=off  show_param=off
      settings: xl_area=[0, 0, 0, 0, 0, 0, 0]
  Delay7 : xbsIndex_r3/Delay  latency=1  reg_retiming=off  explicit_period=on  period=1  en=off  accept_only_valid=off  init_zero=on  dbl_ovrd=off  show_param=off
      settings: xl_area=[0, 0, 0, 0, 0, 0, 0]
  Delay8 : xbsIndex_r3/Delay  latency=1  reg_retiming=off  explicit_period=on  period=1  en=off  accept_only_valid=off  init_zero=on  dbl_ovrd=off  show_param=off
      settings: xl_area=[0, 0, 0, 0, 0, 0, 0]
  Mux : xbsIndex_r3/Mux  inputs=2  precision=Full  arith_type="Signed  (2's comp)"  n_bits=8  bin_pt=2  quantization=Truncate  overflow=Wrap  latency=1  explicit_period=off  period=1  en=off  dbl_ovrd=off  show_param=off  mux_type=off  use_rpm=off  gen_core=off
      settings: xl_area=[0, 0, 0, 0, 0, 0, 0]
  Relational : xbsIndex_r3/Relational  mode=a<b  latency=0  explicit_period=off  period=1  en=off  dbl_ovrd=off  show_param=off
      settings: xl_area=[0, 0, 0, 0, 0, 0, 0]
  delay : Subsystem  BlockChoice=delay_bram
      link override delay_bram: DelayLen=acc_len  bram_latency=bram_latency
      link override delay_bram/Constant2: equ=P=C
      link override delay_slr: DelayLen=acc_len
      settings: AttributesFormatString=%<BlockChoice>  TemplateBlock=casper_library/Delays/delay  MemberBlocks=delay_bram,delay_slr
  dual_pol_cmac : Subsystem
  a_del_out : Outport
  a_ndel_out : Outport  Port=2
  a_end_out : Outport  Port=3
  acc_out : Outport  Port=4
  valid_out : Outport  Port=5
  rst_out : Outport  Port=6
  sync_out : Outport  Port=7
  wires:
  delay/1(Out1) -> Delay3/1
  Mux/1 -> dual_pol_cmac/2(a2)
  Counter/1 -> Relational/1
  Constant/1 -> Relational/2
  Relational/1 -> Convert/1
  Convert/1 -> Mux/1
  rst/1 -> Delay1/1, Counter/1
  a_del/1 -> delay/1(In1)
  dual_pol_cmac/1(acc_out) -> acc_out/1
  acc_in/1 -> dual_pol_cmac/3(acc_in)
  dual_pol_cmac/2(valid_out) -> valid_out/1
  valid_in/1 -> dual_pol_cmac/5(valid_in)
  a_ndel/1 -> Mux/2, Delay7/1
  a_end/1 -> Mux/3, Delay8/1
  Delay3/1 -> dual_pol_cmac/1(a1), a_del_out/1
  Delay7/1 -> a_ndel_out/1
  Delay8/1 -> a_end_out/1
  Delay1/1 -> dual_pol_cmac/4(sync), rst_out/1
  sync1/1 -> sync_out/1

== system b_r309c_med/win_x_engine0/baseline_tap3 ==
  a_del : Inport  Port=1  LatchInput=off
  a_ndel : Inport  Port=2  LatchInput=off
  a_end : Inport  Port=3  LatchInput=off
  acc_in : Inport  Port=4  LatchInput=off
  valid_in : Inport  Port=5  LatchInput=off
  rst : Inport  Port=6  LatchInput=off
  sync1 : Inport  Port=7  LatchInput=off
  Constant : xbsIndex_r3/Constant  const=ant_sep * acc_len  equ=P=C  arith_type=Unsigned  n_bits=ant_bits + bit_growth  bin_pt=0  opselect=C  inp2=PCIN>>17  opr=+  inp1=P  carry=CIN  iostate=0  explicit_period=off  period=1  dbl_ovrd=off
  Convert : xbsIndex_r3/Convert  arith_type=Unsigned  n_bits=1  bin_pt=0  quantization=Truncate  overflow=Wrap  latency=0  explicit_period=off  period=1  dbl_ovrd=off  show_param=off  inserted_by_tool=off  pipeline=off
      settings: xl_area=[0, 0, 0, 0, 0, 0, 0]
  Counter : xbsIndex_r3/Counter  cnt_type=Count Limited  n_bits=ant_bits + bit_growth  bin_pt=0  arith_type=Unsigned  start_count=0  cnt_to=n_ants * acc_len - 1  cnt_by_val=1  operation=Up  explicit_period=off  period=1  load_pin=off  rst=on  en=off  dbl_ovrd=off  show_param=off  use_rpm=on  gen_core=off
      settings: xl_area=[0, 0, 0, 0, 0, 0, 0]
  Delay1 : xbsIndex_r3/Delay  latency=1  reg_retiming=off  explicit_period=off  period=1  en=off  accept_only_valid=off  init_zero=on  dbl_ovrd=off  show_param=off
      settings: xl_area=[0, 0, 0, 0, 0, 0, 0]
  Delay3 : xbsIndex_r3/Delay  latency=1  reg_retiming=off  explicit_period=off  period=1  en=off  accept_only_valid=off  init_zero=on  dbl_ovrd=off  show_param=off
      settings: xl_area=[0, 0, 0, 0, 0, 0, 0]
  Delay7 : xbsIndex_r3/Delay  latency=1  reg_retiming=off  explicit_period=on  period=1  en=off  accept_only_valid=off  init_zero=on  dbl_ovrd=off  show_param=off
      settings: xl_area=[0, 0, 0, 0, 0, 0, 0]
  Delay8 : xbsIndex_r3/Delay  latency=1  reg_retiming=off  explicit_period=on  period=1  en=off  accept_only_valid=off  init_zero=on  dbl_ovrd=off  show_param=off
      settings: xl_area=[0, 0, 0, 0, 0, 0, 0]
  Mux : xbsIndex_r3/Mux  inputs=2  precision=Full  arith_type="Signed  (2's comp)"  n_bits=8  bin_pt=2  quantization=Truncate  overflow=Wrap  latency=1  explicit_period=off  period=1  en=off  dbl_ovrd=off  show_param=off  mux_type=off  use_rpm=off  gen_core=off
      settings: xl_area=[0, 0, 0, 0, 0, 0, 0]
  Relational : xbsIndex_r3/Relational  mode=a<b  latency=0  explicit_period=off  period=1  en=off  dbl_ovrd=off  show_param=off
      settings: xl_area=[0, 0, 0, 0, 0, 0, 0]
  delay : Subsystem  BlockChoice=delay_bram
      link override delay_bram: DelayLen=acc_len  bram_latency=bram_latency
      link override delay_bram/Constant2: equ=P=C
      link override delay_slr: DelayLen=acc_len
      settings: AttributesFormatString=%<BlockChoice>  TemplateBlock=casper_library/Delays/delay  MemberBlocks=delay_bram,delay_slr
  dual_pol_cmac : Subsystem
  a_del_out : Outport
  a_ndel_out : Outport  Port=2
  a_end_out : Outport  Port=3
  acc_out : Outport  Port=4
  valid_out : Outport  Port=5
  rst_out : Outport  Port=6
  sync_out : Outport  Port=7
  wires:
  delay/1(Out1) -> Delay3/1
  Mux/1 -> dual_pol_cmac/2(a2)
  Counter/1 -> Relational/1
  Constant/1 -> Relational/2
  Relational/1 -> Convert/1
  Convert/1 -> Mux/1
  rst/1 -> Delay1/1, Counter/1
  a_del/1 -> delay/1(In1)
  dual_pol_cmac/1(acc_out) -> acc_out/1
  acc_in/1 -> dual_pol_cmac/3(acc_in)
  dual_pol_cmac/2(valid_out) -> valid_out/1
  valid_in/1 -> dual_pol_cmac/5(valid_in)
  a_ndel/1 -> Mux/2, Delay7/1
  a_end/1 -> Mux/3, Delay8/1
  Delay3/1 -> dual_pol_cmac/1(a1), a_del_out/1
  Delay7/1 -> a_ndel_out/1
  Delay8/1 -> a_end_out/1
  Delay1/1 -> dual_pol_cmac/4(sync), rst_out/1
  sync1/1 -> sync_out/1

== system b_r309c_med/win_x_engine0/baseline_tap4 ==
  a_del : Inport  Port=1  LatchInput=off
  a_ndel : Inport  Port=2  LatchInput=off
  a_end : Inport  Port=3  LatchInput=off
  acc_in : Inport  Port=4  LatchInput=off
  valid_in : Inport  Port=5  LatchInput=off
  rst : Inport  Port=6  LatchInput=off
  sync1 : Inport  Port=7  LatchInput=off
  Constant : xbsIndex_r3/Constant  const=ant_sep * acc_len  equ=P=C  arith_type=Unsigned  n_bits=ant_bits + bit_growth  bin_pt=0  opselect=C  inp2=PCIN>>17  opr=+  inp1=P  carry=CIN  iostate=0  explicit_period=off  period=1  dbl_ovrd=off
  Convert : xbsIndex_r3/Convert  arith_type=Unsigned  n_bits=1  bin_pt=0  quantization=Truncate  overflow=Wrap  latency=0  explicit_period=off  period=1  dbl_ovrd=off  show_param=off  inserted_by_tool=off  pipeline=off
      settings: xl_area=[0, 0, 0, 0, 0, 0, 0]
  Counter : xbsIndex_r3/Counter  cnt_type=Count Limited  n_bits=ant_bits + bit_growth  bin_pt=0  arith_type=Unsigned  start_count=0  cnt_to=n_ants * acc_len - 1  cnt_by_val=1  operation=Up  explicit_period=off  period=1  load_pin=off  rst=on  en=off  dbl_ovrd=off  show_param=off  use_rpm=on  gen_core=off
      settings: xl_area=[0, 0, 0, 0, 0, 0, 0]
  Delay1 : xbsIndex_r3/Delay  latency=1  reg_retiming=off  explicit_period=off  period=1  en=off  accept_only_valid=off  init_zero=on  dbl_ovrd=off  show_param=off
      settings: xl_area=[0, 0, 0, 0, 0, 0, 0]
  Delay3 : xbsIndex_r3/Delay  latency=1  reg_retiming=off  explicit_period=off  period=1  en=off  accept_only_valid=off  init_zero=on  dbl_ovrd=off  show_param=off
      settings: xl_area=[0, 0, 0, 0, 0, 0, 0]
  Delay7 : xbsIndex_r3/Delay  latency=1  reg_retiming=off  explicit_period=on  period=1  en=off  accept_only_valid=off  init_zero=on  dbl_ovrd=off  show_param=off
      settings: xl_area=[0, 0, 0, 0, 0, 0, 0]
  Delay8 : xbsIndex_r3/Delay  latency=1  reg_retiming=off  explicit_period=on  period=1  en=off  accept_only_valid=off  init_zero=on  dbl_ovrd=off  show_param=off
      settings: xl_area=[0, 0, 0, 0, 0, 0, 0]
  Mux : xbsIndex_r3/Mux  inputs=2  precision=Full  arith_type="Signed  (2's comp)"  n_bits=8  bin_pt=2  quantization=Truncate  overflow=Wrap  latency=1  explicit_period=off  period=1  en=off  dbl_ovrd=off  show_param=off  mux_type=off  use_rpm=off  gen_core=off
      settings: xl_area=[0, 0, 0, 0, 0, 0, 0]
  Relational : xbsIndex_r3/Relational  mode=a<b  latency=0  explicit_period=off  period=1  en=off  dbl_ovrd=off  show_param=off
      settings: xl_area=[0, 0, 0, 0, 0, 0, 0]
  delay : Subsystem  BlockChoice=delay_bram
      link override delay_bram: DelayLen=acc_len  bram_latency=bram_latency
      link override delay_bram/Constant2: equ=P=C
      link override delay_slr: DelayLen=acc_len
      settings: AttributesFormatString=%<BlockChoice>  TemplateBlock=casper_library/Delays/delay  MemberBlocks=delay_bram,delay_slr
  dual_pol_cmac : Subsystem
  a_del_out : Outport
  a_ndel_out : Outport  Port=2
  a_end_out : Outport  Port=3
  acc_out : Outport  Port=4
  valid_out : Outport  Port=5
  rst_out : Outport  Port=6
  sync_out : Outport  Port=7
  wires:
  delay/1(Out1) -> Delay3/1
  Mux/1 -> dual_pol_cmac/2(a2)
  Counter/1 -> Relational/1
  Constant/1 -> Relational/2
  Relational/1 -> Convert/1
  Convert/1 -> Mux/1
  rst/1 -> Delay1/1, Counter/1
  a_del/1 -> delay/1(In1)
  dual_pol_cmac/1(acc_out) -> acc_out/1
  acc_in/1 -> dual_pol_cmac/3(acc_in)
  dual_pol_cmac/2(valid_out) -> valid_out/1
  valid_in/1 -> dual_pol_cmac/5(valid_in)
  a_ndel/1 -> Mux/2, Delay7/1
  a_end/1 -> Mux/3, Delay8/1
  Delay3/1 -> dual_pol_cmac/1(a1), a_del_out/1
  Delay7/1 -> a_ndel_out/1
  Delay8/1 -> a_end_out/1
  Delay1/1 -> dual_pol_cmac/4(sync), rst_out/1
  sync1/1 -> sync_out/1
